simulink model "controller_Harness_Torque"  (R2023b)
settings: Solver=FixedStepAuto  StartTime=0.0  StopTime=40  FixedStep=1/100  RelTol=1e-3
libraries: simulink x2
settings Model: Creator=Matteo  LastModifiedBy=dadog
settings OptimizationCC: ReuseModelBlockBuffer=off
settings DebuggingCC: SigSpecEnsureSampleTimeMsg=none  UnconnectedInputMsg=warning  UnconnectedOutputMsg=warning  UnconnectedLineMsg=warning
settings ModelReferenceCC: EnableRefExpFcnMdlSchedulingChecks=on
settings RTWCC: DLArmComputeVersion=19.05
settings ConfigComp: CovEnable=on  RecordCoverage=on  CovModelRefEnable=on

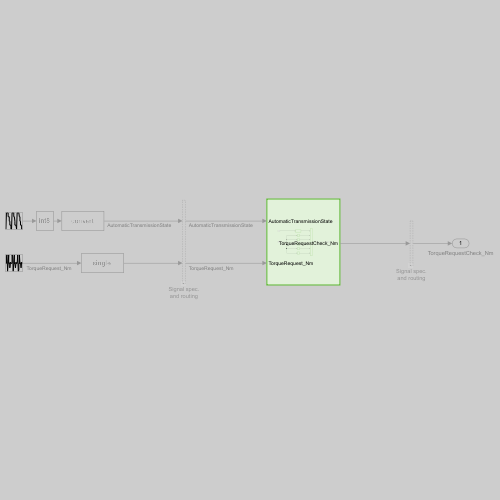
[thumbnail: Simulink's stored preview of the top-level diagram]
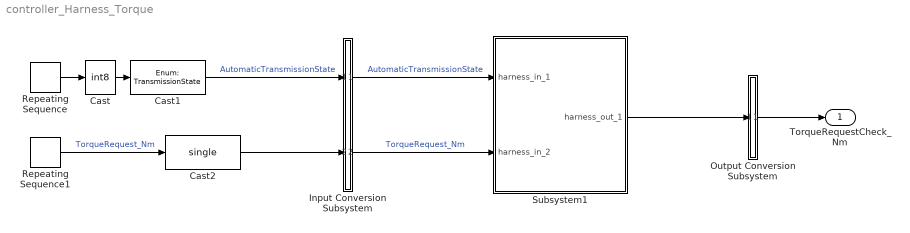
== system controller_Harness_Torque ==
  Cast : DataTypeConversion  OutDataTypeStr=int8  SaturateOnIntegerOverflow=off  RndMeth=Floor
  Cast1 : DataTypeConversion  OutDataTypeStr=Enum: TransmissionState  SaturateOnIntegerOverflow=off  RndMeth=Floor
  Cast2 : DataTypeConversion  OutDataTypeStr=single  SaturateOnIntegerOverflow=off  RndMeth=Floor
  Input Conversion Subsystem : Subsystem  Tag=__SLT_ICS__  Description=|
      | Signal spec.
      | and routing
      settings: AttributesFormatString=%<Description>
  Output Conversion Subsystem : Subsystem  Tag=__SLT_OCS__  Description=|
      | Signal spec.
      | and routing
      settings: AttributesFormatString=%<Description>
  Repeating Sequence : simulink/Sources/Repeating Sequence  rep_seq_t=[0 4 17 18 24 25 27.5 28 36 37 40]  rep_seq_y=[0 4 4 3 3 2 2 1 1 0 0]
  Repeating Sequence1 : simulink/Sources/Repeating Sequence  rep_seq_t=[0 4 6 7 8 12 13 14 17 18 20 22 23 24 25 26 27 28 30 35 36 37 38 39 40]  rep_seq_y=[0 0 80 90 80 -80 -90 -80 0 0 90 0 -10 0 0 4 -4 0 -50 10 0 0 5 -5 0]
  Subsystem1 : Subsystem  Tag=__SL_testing_harness_stub_
  TorqueRequestCheck_Nm : Outport
  wires:
  Cast1/1 -> Input Conversion Subsystem/1(Inport_1)  "AutomaticTransmissionState"
  Repeating Sequence1/1 -> Cast2/1  "TorqueRequest_Nm"
  Output Conversion Subsystem/1(Outport_1) -> TorqueRequestCheck_Nm/1
  Input Conversion Subsystem/1(Outport_1) -> Subsystem1/1(harness_in_1)  "AutomaticTransmissionState"
  Input Conversion Subsystem/2(Outport_2) -> Subsystem1/2(harness_in_2)  "TorqueRequest_Nm"
  Subsystem1/1(harness_out_1) -> Output Conversion Subsystem/1(Inport_1)
  Cast/1 -> Cast1/1
  Repeating Sequence/1 -> Cast/1
  Cast2/1 -> Input Conversion Subsystem/2(Inport_2)

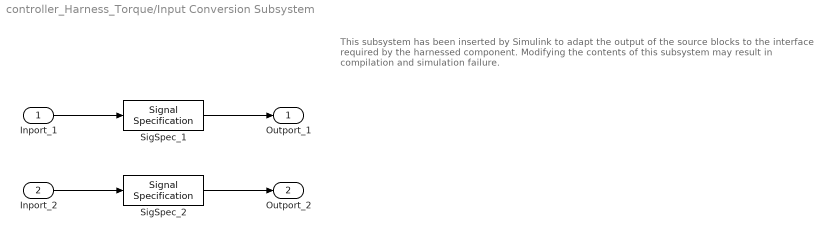
== system controller_Harness_Torque/Input Conversion Subsystem ==
  note: This subsystem has been inserted by Simulink to adapt the output of the source blocks to the interface required by the harnessed component.
      |  Modifying the contents of this subsystem may result in compilation and simulation failure.
  Inport_1 : Inport
  Inport_2 : Inport  Port=2
  SigSpec_1 : SignalSpecification  OutDataTypeStr=Enum: TransmissionState  Dimensions=[1]  SampleTime=0.01
  SigSpec_2 : SignalSpecification  OutDataTypeStr=single  Dimensions=[1]  SampleTime=0.01
  Outport_1 : Outport
  Outport_2 : Outport  Port=2
  wires:
  SigSpec_1/1 -> Outport_1/1
  Inport_1/1 -> SigSpec_1/1
  SigSpec_2/1 -> Outport_2/1
  Inport_2/1 -> SigSpec_2/1

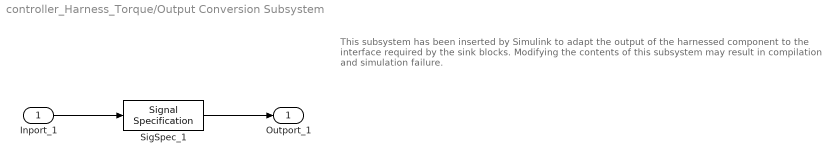
== system controller_Harness_Torque/Output Conversion Subsystem ==
  note: This subsystem has been inserted by Simulink to adapt the output of the harnessed component to the interface required by the sink blocks.
      |  Modifying the contents of this subsystem may result in compilation and simulation failure.
  Inport_1 : Inport
  SigSpec_1 : SignalSpecification  OutDataTypeStr=single  Dimensions=[1]  SampleTime=0.01
  Outport_1 : Outport
  wires:
  Inport_1/1 -> SigSpec_1/1
  SigSpec_1/1 -> Outport_1/1

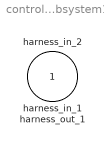
== system controller_Harness_Torque/Subsystem1 ==
  harness_in_1 : Inport
  harness_in_2 : Inport  Port=2
  harness_out_1 : Outport
